simulink model "sampleModel112"  (R2021b)
settings: Solver=VariableStepAuto  StartTime=0.0  StopTime=10.0  RelTol=1e-3
libraries: simulink x8
settings Model: Creator=user  LastModifiedBy=user

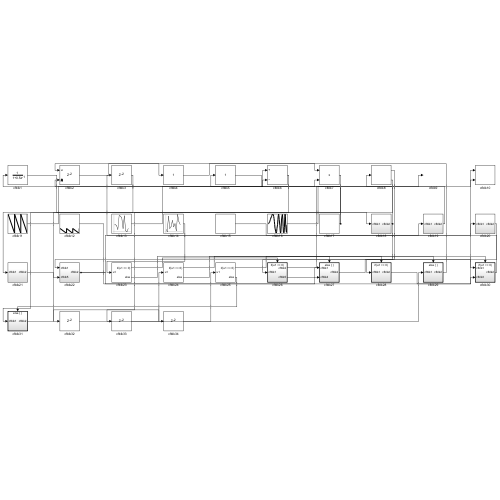
[thumbnail: Simulink's stored preview of the top-level diagram]
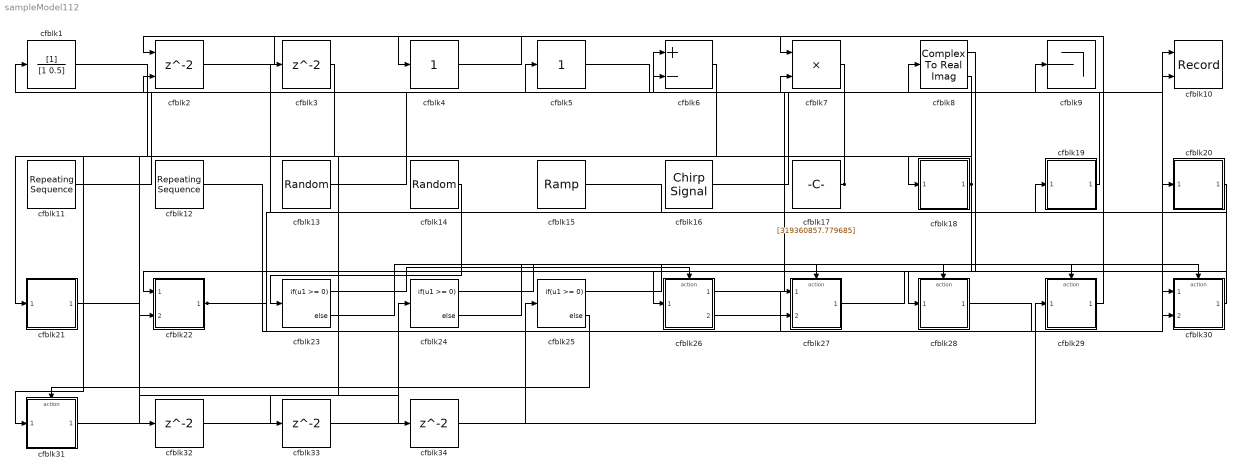
== system sampleModel112 ==
  cfblk1 : DiscreteFilter  SampleTime=1
  cfblk10 : Record  FileSettingsInternal="{\"entries\":[{\"content\":{\"excelSettings\":{\"content\":{},\"type\":\"Streamout.ExcelSettings\"}},\"type\":\"Streamout.FileSettingStorage\",\"uuid\":\"e7662b0d-9788-4241-b231-2d1bc495edf1\"}],\"packageUris\":[\"http://schema.mathworks.com/mf0/streamout_blocks/R2020a\"],\"version\":\"1.0\"}"  Layout=[1 1]  SignalsInternal="{\"entries\":[{\"content\":{\"signals\":[{\"content\":{\"blockPath\":[\"sampleModel112/cfblk10\"],\"channel\":[],\"dimensions\":[1],\"domain\":\"sampleModel112/cfblk10\",\"lineColor\":\"#a2142f\",\"plots\":[1],\"port\":1,\"sid\":[\"\"],\"signalID\":3893,\"signalName\":\"cfblk12\"},\"type\":\"RecordBlkView.Signal\",\"uuid\":\"768b1969-7b99-49bf-8f29-881fa0714196\"},{\"content\":{\"blockPath\":[\"sampleModel112/cfblk10\"],\"channel\":[],\"dimensions\":[1],\"domain\":\"sampleModel112/cfblk10\",\"lineColor\":\"#139fff\",\"plots\":[1],\"port\":2,\"sid\":[\"\"],\"signalID\":3897,\"signalName\":\"cfblk26:1\"},\"type\":\"RecordBlkView.Signal\",\"uuid\":\"19a3c30b-6c93-4a22-a47f-53b55a2b8fe2\"}]},\"type\":\"RecordBlkView.InputSignals\",\"uuid\":\"6b4ad7aa-f3ae-4b35-a691-488c5842ed91\"}],\"packageUris\":[\"http://schema.mathworks.com/mf0/streamout_blocks/R2020a\"],\"version\":\"1.0\"}"  VisualizationBindings="{\"xyplotplugin\":{\"info\":[{\"series\":[{\"bindingParametersList\":[{\"parameter\":\"X-Axis\",\"signalID\":3893,\"signalName\":\"cfblk12\"},{\"parameter\":\"Y-Axis\",\"signalID\":3897,\"signalName\":\"cfblk26:1\"}],\"seriesID\":16983}],\"subplotID\":1}]}}"  CompatibilityTag=XY
  cfblk11 : simulink/Sources/Repeating Sequence  rep_seq_t=[0 2]  rep_seq_y=[651977519.239512, 445399278.187059]
  cfblk12 : simulink/Sources/Repeating Sequence  rep_seq_t=[0 2]  rep_seq_y=[-638354459.572029, -857079308.126003]
  cfblk13 : RandomNumber  Mean=[-82983.500332]  Variance=[79082.987878]  Seed=[308454848.000000]  SampleTime=0.1
  cfblk14 : UniformRandomNumber  Minimum=[-3368545703.776334]  Maximum=[7952096108.975738]  Seed=[61725340.000000]  SampleTime=0.1
  cfblk15 : simulink/Sources/Ramp  slope=[1247.753617]  start=[41.930011]  InitialOutput=[-89359.293500]
  cfblk16 : simulink/Sources/Chirp Signal  f1=[-640750665.714521]  T=[-979471842.197449]  f2=[817802052.682605]
  cfblk17 : Constant  Value=[319360857.779685]  SampleTime=1
  cfblk18 : Subsystem
  cfblk19 : Subsystem
  cfblk2 : Delay  ShowEnablePort=on  SampleTime=1
      settings: InputPortMap=u0,e6
  cfblk20 : Subsystem
  cfblk21 : Subsystem
  cfblk22 : Subsystem
  cfblk23 : If  IfExpression=u1 >= 0  SampleTime=1
  cfblk24 : If  IfExpression=u1 >= 0  SampleTime=1
  cfblk25 : If  IfExpression=u1 >= 0  SampleTime=1
  cfblk26 : Subsystem  TreatAsAtomicUnit=on
  cfblk27 : Subsystem  TreatAsAtomicUnit=on
  cfblk28 : Subsystem  TreatAsAtomicUnit=on
  cfblk29 : Subsystem  TreatAsAtomicUnit=on
  cfblk{3,32..34} (4 alike) : Delay  SampleTime=1
  cfblk30 : Subsystem  TreatAsAtomicUnit=on
  cfblk31 : Subsystem  TreatAsAtomicUnit=on
  cfblk4 : simulink/Math Operations/Slider Gain  gain=1  low=0  high=2
  cfblk5 : simulink/Math Operations/Slider Gain  gain=1  low=0  high=2
  cfblk6 : Sum  Inputs=+-
  cfblk7 : Product
  cfblk8 : ComplexToRealImag
  cfblk9 : Terminator
  wires:
  cfblk14/1 -> cfblk23/1
  cfblk16/1 -> cfblk9/1
  cfblk11/1 -> cfblk6/1
  cfblk29/1(cfblk2) -> cfblk2/1
  cfblk3/1 -> cfblk21/1(cfblk1)
  cfblk15/1 -> cfblk19/1(cfblk1)
  cfblk12/1 -> cfblk10/1
  cfblk26/1(cfblk2) -> cfblk10/2
  cfblk1/1 -> cfblk18/1(cfblk1)
  cfblk19/1(cfblk2) -> cfblk5/1
  cfblk4/1 -> cfblk7/1
  cfblk18/1(cfblk2) -> cfblk28/1(cfblk1), cfblk8/1
  cfblk20/1(cfblk2) -> cfblk26/1(cfblk1)
  cfblk17/1 -> cfblk2/2, cfblk1/1
  cfblk2/1 -> cfblk4/1
  cfblk13/1 -> cfblk6/2
  cfblk30/1(cfblk2) -> cfblk3/1
  cfblk26/2(cfblk5) -> cfblk27/1(cfblk1)
  cfblk8/1 -> cfblk22/1(cfblk1)
  cfblk6/1 -> cfblk22/2(cfblk5)
  cfblk22/1(cfblk2) -> cfblk27/2(cfblk4), cfblk20/1(cfblk1)
  cfblk27/1(cfblk2) -> cfblk30/1(cfblk1)
  cfblk8/2 -> cfblk31/1(cfblk1)
  cfblk5/1 -> cfblk7/2
  cfblk28/1(cfblk2) -> cfblk30/2(cfblk3)
  cfblk23/1 -> cfblk26/Action
  cfblk23/2 -> cfblk27/Action
  cfblk24/1 -> cfblk28/Action
  cfblk24/2 -> cfblk29/Action
  cfblk25/1 -> cfblk30/Action
  cfblk25/2 -> cfblk31/Action
  cfblk21/1(cfblk2) -> cfblk32/1
  cfblk32/1 -> cfblk24/1
  cfblk7/1 -> cfblk33/1
  cfblk33/1 -> cfblk25/1
  cfblk31/1(cfblk2) -> cfblk34/1
  cfblk34/1 -> cfblk29/1(cfblk1)

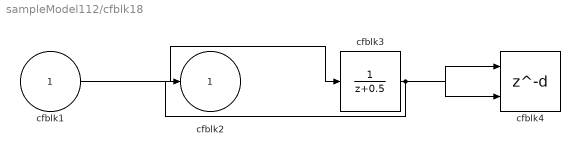
== system sampleModel112/cfblk18 ==
  cfblk1 : Inport
  cfblk3 : DiscreteTransferFcn  SampleTime=1
  cfblk4 : Delay  DelayLengthSource=Input port  SampleTime=1
      settings: InputPortMap=u0,p1
  cfblk2 : Outport
  wires:
  cfblk1/1 -> cfblk3/1
  cfblk3/1 -> cfblk2/1, cfblk4/1, cfblk4/2

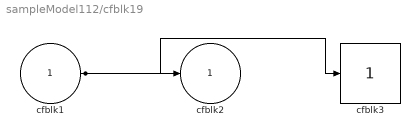
== system sampleModel112/cfblk19 ==
  cfblk1 : Inport
  cfblk3 : simulink/Math Operations/Slider Gain  gain=1  low=0  high=2
  cfblk2 : Outport
  wires:
  cfblk1/1 -> cfblk2/1, cfblk3/1

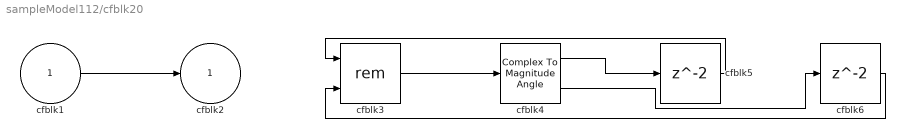
== system sampleModel112/cfblk20 ==
  cfblk1 : Inport
  cfblk3 : Math  Operator=rem  SaturateOnIntegerOverflow=on
  cfblk4 : ComplexToMagnitudeAngle
  cfblk5 : Delay  SampleTime=1
  cfblk6 : Delay  SampleTime=1
  cfblk2 : Outport
  wires:
  cfblk1/1 -> cfblk2/1
  cfblk3/1 -> cfblk4/1
  cfblk4/1 -> cfblk5/1
  cfblk5/1 -> cfblk3/1
  cfblk4/2 -> cfblk6/1
  cfblk6/1 -> cfblk3/2

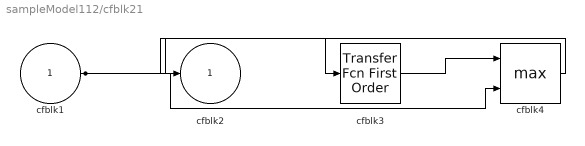
== system sampleModel112/cfblk21 ==
  cfblk1 : Inport
  cfblk3 : simulink/Discrete/Transfer Fcn First Order  PoleZ=0.95  ICPrevOutput=0.0  DoSatur=off
  cfblk4 : MinMax  Function=max  Inputs=2
  cfblk2 : Outport
  wires:
  cfblk3/1 -> cfblk4/1
  cfblk1/1 -> cfblk4/2, cfblk3/1
  cfblk4/1 -> cfblk2/1

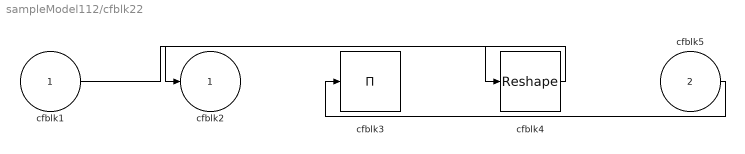
== system sampleModel112/cfblk22 ==
  cfblk1 : Inport
  cfblk5 : Inport  Port=2
  cfblk3 : Product  Inputs=*
  cfblk4 : Reshape
  cfblk2 : Outport
  wires:
  cfblk4/1 -> cfblk2/1
  cfblk5/1 -> cfblk3/1
  cfblk1/1 -> cfblk4/1

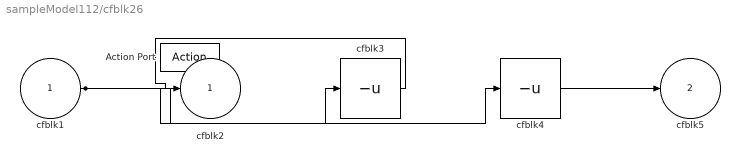
== system sampleModel112/cfblk26 ==
  cfblk1 : Inport
  Action Port : ActionPort  ActionPortLabel=if(u1 >= 0)
  cfblk3 : UnaryMinus
  cfblk4 : UnaryMinus
  cfblk2 : Outport
  cfblk5 : Outport  Port=2
  wires:
  cfblk1/1 -> cfblk4/1, cfblk3/1
  cfblk3/1 -> cfblk2/1
  cfblk4/1 -> cfblk5/1

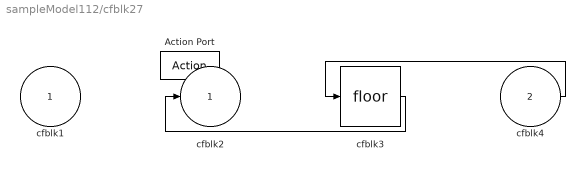
== system sampleModel112/cfblk27 ==
  cfblk1 : Inport
  cfblk4 : Inport  Port=2
  Action Port : ActionPort  ActionPortLabel=else
  cfblk3 : Rounding
  cfblk2 : Outport
  wires:
  cfblk3/1 -> cfblk2/1
  cfblk4/1 -> cfblk3/1

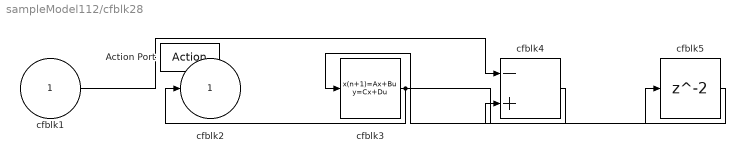
== system sampleModel112/cfblk28 ==
  cfblk1 : Inport
  Action Port : ActionPort  ActionPortLabel=if(u1 >= 0)
  cfblk3 : DiscreteStateSpace  SampleTime=-1
  cfblk4 : Sum  Inputs=-+
  cfblk5 : Delay
  cfblk2 : Outport
  wires:
  cfblk3/1 -> cfblk2/1, cfblk5/1
  cfblk1/1 -> cfblk4/1
  cfblk4/1 -> cfblk3/1
  cfblk5/1 -> cfblk4/2

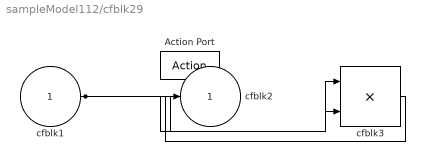
== system sampleModel112/cfblk29 ==
  cfblk1 : Inport
  Action Port : ActionPort  ActionPortLabel=else
  cfblk3 : Product
  cfblk2 : Outport
  wires:
  cfblk1/1 -> cfblk3/1, cfblk3/2
  cfblk3/1 -> cfblk2/1

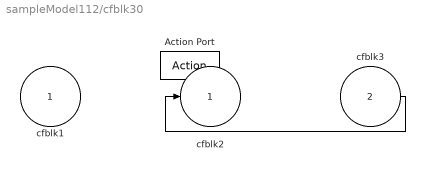
== system sampleModel112/cfblk30 ==
  cfblk1 : Inport
  cfblk3 : Inport  Port=2
  Action Port : ActionPort  ActionPortLabel=if(u1 >= 0)
  cfblk2 : Outport
  wires:
  cfblk3/1 -> cfblk2/1

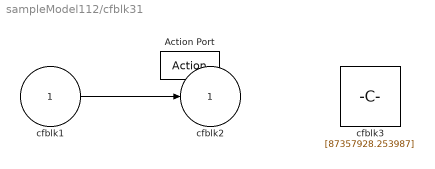
== system sampleModel112/cfblk31 ==
  cfblk1 : Inport
  Action Port : ActionPort  ActionPortLabel=else
  cfblk3 : Constant  Value=[87357928.253987]  SampleTime=1
  cfblk2 : Outport
  wires:
  cfblk1/1 -> cfblk2/1
